simulink model "DiffToSingle"  (R2025b)
settings: Solver=VariableStepAuto  StartTime=0.0  StopTime=0.5e-3  RelTol=1e-3
InitFcn:
  | % -------------------------------------------------------------------------
  | %  [1.4] Diferencial a Single-Ended
  | % -------------------------------------------------------------------------
  | Rab      = 40e3;   % (Ohm)
  | Ra_dse   = 10e3;   % (Ohm)
  | Rb_dse   = 490e3;  % (Ohm)
  | Rlow_dse = 1e6;    % (Ohm)
  | Clow_dse = 11e-12; % (F)
  | 
  | Vmin = -1e3;
  | Vmax = 1e3;
  | SR   = 4.3e6;
  | Rin  = 35e6;
  | Rout = 20;
  | Gain = 10^(90/20);
  | BW   = 8e6/Gain;
StartFcn:
  | % -------------------------------------------------------------------------
  | %  [1.4] Diferencial a Single-Ended
  | % -------------------------------------------------------------------------
  | Rab      = 40e3;   % (Ohm)
  | Ra_dse   = 10e3;   % (Ohm)
  | Rb_dse   = 490e3;  % (Ohm)
  | Rlow_dse = 1e6;    % (Ohm)
  | Clow_dse = 11e-12; % (F)
  | 
  | Vmin = -1e3;
  | Vmax = 1e3;
  | SR   = 4.3e6;
  | Rin  = 35e6;
  | Rout = 20;
  | Gain = 10^(90/20);
  | BW   = 8e6/Gain;
settings Model: Creator=elias  LastModifiedBy=elias

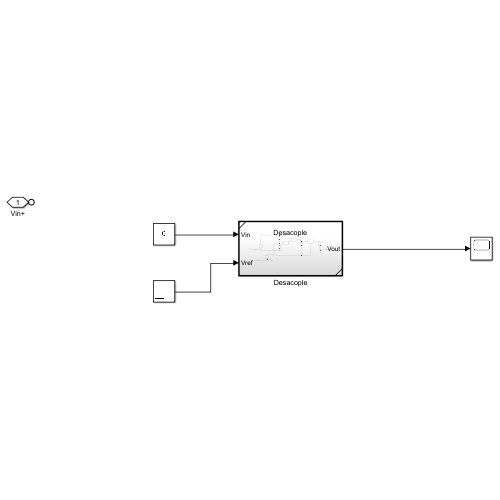
[thumbnail: Simulink's stored preview of the top-level diagram]
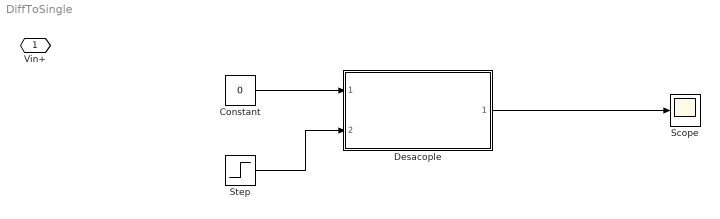
== system DiffToSingle ==
  Constant : Constant  Value=0
  Desacople : Subsystem  TreatAsAtomicUnit=on  ReferencedSubsystem=Desacople
  Scope : Scope
      settings: ActiveDisplayYMinimum=-0.84101019077036476  ActiveDisplayYMaximum=1.1659121758460447
  Step : Step  Time=0  SampleTime=0
  Vin+ : PMIOPort  Side=Left
  wires:
  Step/1 -> Desacople/2
  Constant/1 -> Desacople/1
  Desacople/1 -> Scope/1
